simulink model "ensembleSNN_simulink"  (R2019a)
settings: Solver=FixedStepAuto  StartTime=0.0  StopTime=12  FixedStep=0.001  RelTol=1e-3
libraries: simulink x2, dspsigops x1
(part 1 of 3)
settings Model: Creator=40129232  LastModifiedBy=40175607
settings DataIOCC: ReturnWorkspaceOutputs=off
settings OptimizationCC: LifeSpan=inf
settings DebuggingCC: SFExecutionAtInitializationDiag=none  ArithmeticOperatorsInVariantConditions=warning
settings SFSimCC: SimUseLocalCustomCode=off
settings RTWCC: RTWUseLocalCustomCode=off
settings CodeAppCC: StateflowObjectComments=on

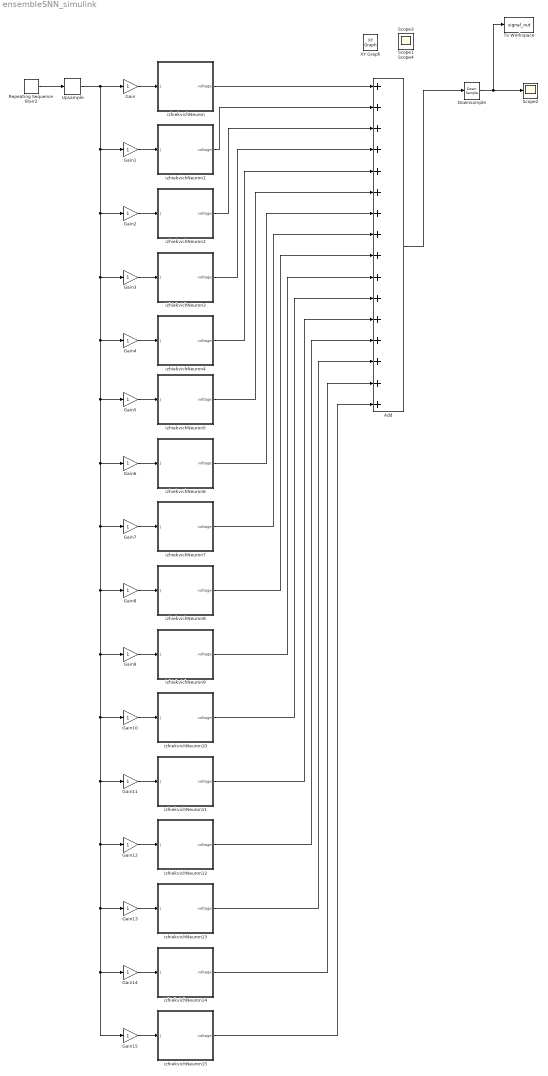
== system ensembleSNN_simulink ==
  Add : Sum  Inputs=++++++++++++++++
  Downsample : DownSample  N=12  phase=9  RateOptions=Allow multirate processing
  Gain{,1..15} (16 alike) : Gain
  Repeating Sequence Stair2 : simulink/Sources/Repeating Sequence Stair  OutValues=[40.37, 52.35, 62.17, 70.19, 76.75].'  tsamp=0.012  OutMin=[]  OutMax=[]  OutDataTypeStr=double  OutputDataTypeScalingMode=double  OutDataType=fixdt(0,8)  ConRadixGroup=Best Precision: Vector-wise  OutScaling=2^-12
  Scope{1..4} (4 alike) : Scope
  To Workspace : ToWorkspace  VariableName=signal_out  SampleTime=-1
  Upsample : dspsigops/Upsample  N=12  phase=0  RateOptions=Allow multirate processing  ic=0  mode=Unused parameter value
  izhiekvichNeuron : Subsystem
  izhiekvichNeuron1 : Subsystem
  izhiekvichNeuron10 : Subsystem
  izhiekvichNeuron11 : Subsystem
  izhiekvichNeuron12 : Subsystem
  izhiekvichNeuron13 : Subsystem
  izhiekvichNeuron14 : Subsystem
  izhiekvichNeuron15 : Subsystem
  izhiekvichNeuron2 : Subsystem
  izhiekvichNeuron3 : Subsystem
  izhiekvichNeuron4 : Subsystem
  izhiekvichNeuron5 : Subsystem
  izhiekvichNeuron6 : Subsystem
  izhiekvichNeuron7 : Subsystem
  izhiekvichNeuron8 : Subsystem
  izhiekvichNeuron9 : Subsystem
  XY Graph : simulink/Sinks/XY Graph  IOType=viewer  xmin=-1  xmax=1  ymin=-1  ymax=1  st=-1
  wires:
  Repeating Sequence Stair2/1 -> Upsample/1
  Downsample/1 -> To Workspace/1, Scope2/1
  Upsample/1 -> Gain3/1, Gain5/1, Gain6/1, Gain9/1, Gain11/1, Gain12/1, Gain15/1, Gain14/1, Gain13/1, Gain10/1, Gain8/1, Gain7/1, Gain4/1, Gain2/1, Gain1/1, Gain/1
  Gain/1 -> izhiekvichNeuron/1(J)
  Add/1 -> Downsample/1
  izhiekvichNeuron/1(voltage) -> Add/1
  izhiekvichNeuron15/1(voltage) -> Add/16
  izhiekvichNeuron14/1(voltage) -> Add/15
  izhiekvichNeuron13/1(voltage) -> Add/14
  izhiekvichNeuron12/1(voltage) -> Add/13
  izhiekvichNeuron11/1(voltage) -> Add/12
  izhiekvichNeuron10/1(voltage) -> Add/11
  izhiekvichNeuron9/1(voltage) -> Add/10
  izhiekvichNeuron8/1(voltage) -> Add/9
  izhiekvichNeuron7/1(voltage) -> Add/8
  izhiekvichNeuron6/1(voltage) -> Add/7
  izhiekvichNeuron5/1(voltage) -> Add/6
  izhiekvichNeuron4/1(voltage) -> Add/5
  izhiekvichNeuron3/1(voltage) -> Add/4
  izhiekvichNeuron2/1(voltage) -> Add/3
  izhiekvichNeuron1/1(voltage) -> Add/2
  Gain1/1 -> izhiekvichNeuron1/1(J)
  Gain2/1 -> izhiekvichNeuron2/1(J)
  Gain3/1 -> izhiekvichNeuron3/1(J)
  Gain4/1 -> izhiekvichNeuron4/1(J)
  Gain5/1 -> izhiekvichNeuron5/1(J)
  Gain6/1 -> izhiekvichNeuron6/1(J)
  Gain7/1 -> izhiekvichNeuron7/1(J)
  Gain8/1 -> izhiekvichNeuron8/1(J)
  Gain9/1 -> izhiekvichNeuron9/1(J)
  Gain10/1 -> izhiekvichNeuron10/1(J)
  Gain11/1 -> izhiekvichNeuron11/1(J)
  Gain12/1 -> izhiekvichNeuron12/1(J)
  Gain13/1 -> izhiekvichNeuron13/1(J)
  Gain14/1 -> izhiekvichNeuron14/1(J)
  Gain15/1 -> izhiekvichNeuron15/1(J)

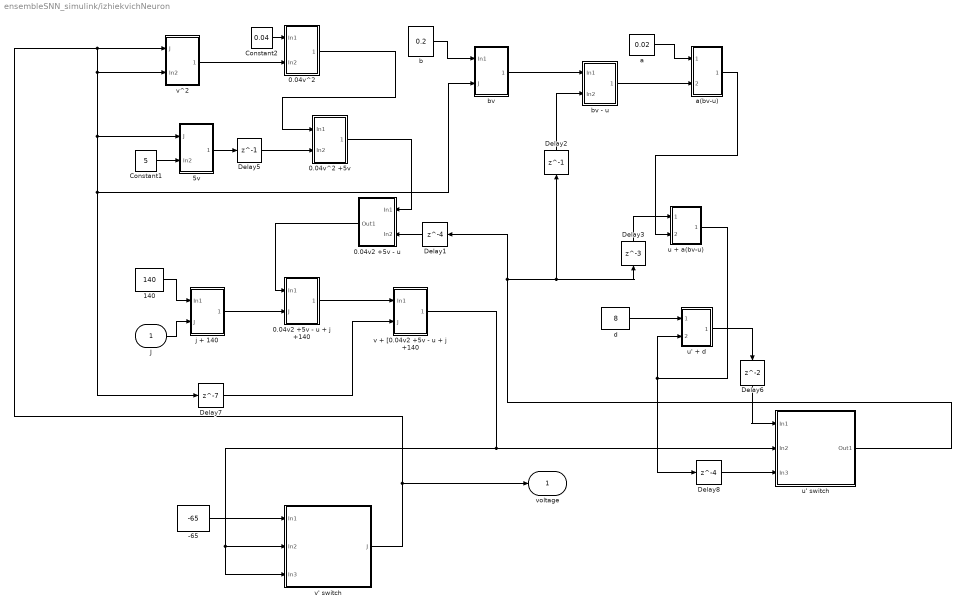
== system ensembleSNN_simulink/izhiekvichNeuron ==
  J : Inport
  -65 : Constant  Value=-65
  0.04v2 +5v - u : Subsystem
  0.04v2 +5v - u + j +140 : Subsystem
  0.04v^2 : Subsystem
  0.04v^2 +5v : Subsystem
  140 : Constant  Value=140
  5v : Subsystem
  Constant1 : Constant  Value=5
  Constant2 : Constant  Value=0.04
  Delay1 : Delay  DelayLength=4
  Delay2 : Delay  DelayLength=1
  Delay3 : Delay  DelayLength=3
  Delay5 : Delay  DelayLength=1
  Delay6 : Delay
  Delay7 : Delay  DelayLength=7
  Delay8 : Delay  DelayLength=4
  a : Constant  Value=0.02
  a(bv-u) : Subsystem
  b : Constant  Value=0.2
  bv : Subsystem
  bv - u : Subsystem
  d : Constant  Value=8
  j + 140 : Subsystem
  u + a(bv-u) : Subsystem
  u' + d : Subsystem
  u' switch : Subsystem
  v + [0.04v2 +5v - u + j +140 : Subsystem
  v' switch : Subsystem
  v^2 : Subsystem
  voltage : Outport
  wires:
  d/1 -> u' + d/1(In1)
  Constant1/1 -> 5v/2(In2)
  Constant2/1 -> 0.04v^2/1(In1)
  140/1 -> j + 140/1(In1)
  -65/1 -> v' switch/1(In1)
  b/1 -> bv/1(In1)
  a/1 -> a(bv-u)/1(In1)
  5v/1(Out1) -> Delay5/1
  J/1 -> j + 140/2(J)
  j + 140/1(Out1) -> 0.04v2 +5v - u + j +140/2(J)
  u' + d/1(Out1) -> Delay6/1
  u' switch/1(Out1) -> Delay1/1, Delay3/1, Delay2/1
  Delay1/1 -> 0.04v2 +5v - u/2(In2)
  Delay2/1 -> bv - u/2(In2)
  Delay3/1 -> u + a(bv-u)/1(In1)
  v' switch/1(J) -> v^2/1(J), v^2/2(In2), 5v/1(J), bv/2(J), Delay7/1, voltage/1
  Delay7/1 -> v + [0.04v2 +5v - u + j +140/2(J)
  v^2/1(Out1) -> 0.04v^2/2(In2)
  Delay5/1 -> 0.04v^2 +5v/2(In2)
  bv/1(Out1) -> bv - u/1(In1)
  0.04v^2/1(Out1) -> 0.04v^2 +5v/1(In1)
  bv - u/1(Out1) -> a(bv-u)/2(In2)
  0.04v^2 +5v/1(Out1) -> 0.04v2 +5v - u/1(In1)
  0.04v2 +5v - u/1(Out1) -> 0.04v2 +5v - u + j +140/1(In1)
  0.04v2 +5v - u + j +140/1(Out1) -> v + [0.04v2 +5v - u + j +140/1(In1)
  v + [0.04v2 +5v - u + j +140/1(Out1) -> u' switch/2(In2), v' switch/3(In3), v' switch/2(In2)
  a(bv-u)/1(Out1) -> u + a(bv-u)/2(In2)
  u + a(bv-u)/1(Out1) -> u' + d/2(In2), Delay8/1
  Delay8/1 -> u' switch/3(In3)
  Delay6/1 -> u' switch/1(In1)

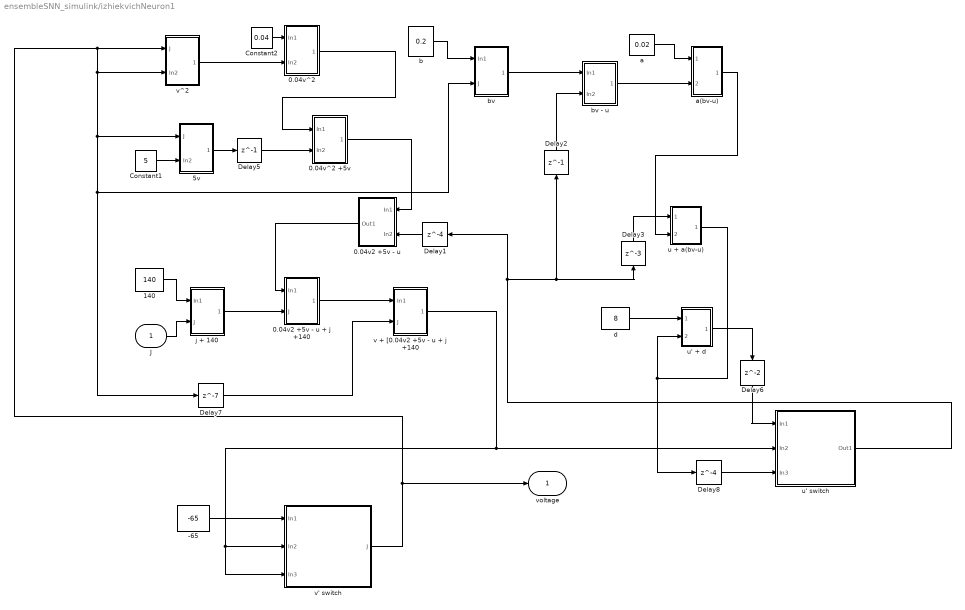
== system ensembleSNN_simulink/izhiekvichNeuron1 ==
  J : Inport
  -65 : Constant  Value=-65
  0.04v2 +5v - u : Subsystem
  0.04v2 +5v - u + j +140 : Subsystem
  0.04v^2 : Subsystem
  0.04v^2 +5v : Subsystem
  140 : Constant  Value=140
  5v : Subsystem
  Constant1 : Constant  Value=5
  Constant2 : Constant  Value=0.04
  Delay1 : Delay  DelayLength=4
  Delay2 : Delay  DelayLength=1
  Delay3 : Delay  DelayLength=3
  Delay5 : Delay  DelayLength=1
  Delay6 : Delay
  Delay7 : Delay  DelayLength=7
  Delay8 : Delay  DelayLength=4
  a : Constant  Value=0.02
  a(bv-u) : Subsystem
  b : Constant  Value=0.2
  bv : Subsystem
  bv - u : Subsystem
  d : Constant  Value=8
  j + 140 : Subsystem
  u + a(bv-u) : Subsystem
  u' + d : Subsystem
  u' switch : Subsystem
  v + [0.04v2 +5v - u + j +140 : Subsystem
  v' switch : Subsystem
  v^2 : Subsystem
  voltage : Outport
  wires:
  d/1 -> u' + d/1(In1)
  Constant1/1 -> 5v/2(In2)
  Constant2/1 -> 0.04v^2/1(In1)
  140/1 -> j + 140/1(In1)
  -65/1 -> v' switch/1(In1)
  b/1 -> bv/1(In1)
  a/1 -> a(bv-u)/1(In1)
  5v/1(Out1) -> Delay5/1
  J/1 -> j + 140/2(J)
  j + 140/1(Out1) -> 0.04v2 +5v - u + j +140/2(J)
  u' + d/1(Out1) -> Delay6/1
  u' switch/1(Out1) -> Delay1/1, Delay3/1, Delay2/1
  Delay1/1 -> 0.04v2 +5v - u/2(In2)
  Delay2/1 -> bv - u/2(In2)
  Delay3/1 -> u + a(bv-u)/1(In1)
  v' switch/1(J) -> v^2/1(J), v^2/2(In2), 5v/1(J), bv/2(J), Delay7/1, voltage/1
  Delay7/1 -> v + [0.04v2 +5v - u + j +140/2(J)
  v^2/1(Out1) -> 0.04v^2/2(In2)
  Delay5/1 -> 0.04v^2 +5v/2(In2)
  bv/1(Out1) -> bv - u/1(In1)
  0.04v^2/1(Out1) -> 0.04v^2 +5v/1(In1)
  bv - u/1(Out1) -> a(bv-u)/2(In2)
  0.04v^2 +5v/1(Out1) -> 0.04v2 +5v - u/1(In1)
  0.04v2 +5v - u/1(Out1) -> 0.04v2 +5v - u + j +140/1(In1)
  0.04v2 +5v - u + j +140/1(Out1) -> v + [0.04v2 +5v - u + j +140/1(In1)
  v + [0.04v2 +5v - u + j +140/1(Out1) -> u' switch/2(In2), v' switch/3(In3), v' switch/2(In2)
  a(bv-u)/1(Out1) -> u + a(bv-u)/2(In2)
  u + a(bv-u)/1(Out1) -> u' + d/2(In2), Delay8/1
  Delay8/1 -> u' switch/3(In3)
  Delay6/1 -> u' switch/1(In1)

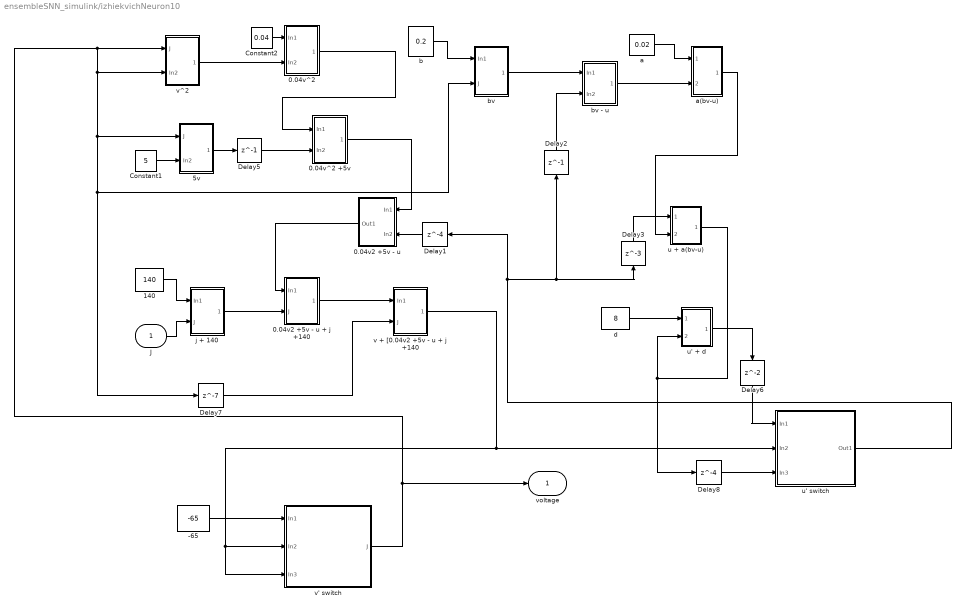
== system ensembleSNN_simulink/izhiekvichNeuron10 ==
  J : Inport
  -65 : Constant  Value=-65
  0.04v2 +5v - u : Subsystem
  0.04v2 +5v - u + j +140 : Subsystem
  0.04v^2 : Subsystem
  0.04v^2 +5v : Subsystem
  140 : Constant  Value=140
  5v : Subsystem
  Constant1 : Constant  Value=5
  Constant2 : Constant  Value=0.04
  Delay1 : Delay  DelayLength=4
  Delay2 : Delay  DelayLength=1
  Delay3 : Delay  DelayLength=3
  Delay5 : Delay  DelayLength=1
  Delay6 : Delay
  Delay7 : Delay  DelayLength=7
  Delay8 : Delay  DelayLength=4
  a : Constant  Value=0.02
  a(bv-u) : Subsystem
  b : Constant  Value=0.2
  bv : Subsystem
  bv - u : Subsystem
  d : Constant  Value=8
  j + 140 : Subsystem
  u + a(bv-u) : Subsystem
  u' + d : Subsystem
  u' switch : Subsystem
  v + [0.04v2 +5v - u + j +140 : Subsystem
  v' switch : Subsystem
  v^2 : Subsystem
  voltage : Outport
  wires:
  d/1 -> u' + d/1(In1)
  Constant1/1 -> 5v/2(In2)
  Constant2/1 -> 0.04v^2/1(In1)
  140/1 -> j + 140/1(In1)
  -65/1 -> v' switch/1(In1)
  b/1 -> bv/1(In1)
  a/1 -> a(bv-u)/1(In1)
  5v/1(Out1) -> Delay5/1
  J/1 -> j + 140/2(J)
  j + 140/1(Out1) -> 0.04v2 +5v - u + j +140/2(J)
  u' + d/1(Out1) -> Delay6/1
  u' switch/1(Out1) -> Delay1/1, Delay3/1, Delay2/1
  Delay1/1 -> 0.04v2 +5v - u/2(In2)
  Delay2/1 -> bv - u/2(In2)
  Delay3/1 -> u + a(bv-u)/1(In1)
  v' switch/1(J) -> v^2/1(J), v^2/2(In2), 5v/1(J), bv/2(J), Delay7/1, voltage/1
  Delay7/1 -> v + [0.04v2 +5v - u + j +140/2(J)
  v^2/1(Out1) -> 0.04v^2/2(In2)
  Delay5/1 -> 0.04v^2 +5v/2(In2)
  bv/1(Out1) -> bv - u/1(In1)
  0.04v^2/1(Out1) -> 0.04v^2 +5v/1(In1)
  bv - u/1(Out1) -> a(bv-u)/2(In2)
  0.04v^2 +5v/1(Out1) -> 0.04v2 +5v - u/1(In1)
  0.04v2 +5v - u/1(Out1) -> 0.04v2 +5v - u + j +140/1(In1)
  0.04v2 +5v - u + j +140/1(Out1) -> v + [0.04v2 +5v - u + j +140/1(In1)
  v + [0.04v2 +5v - u + j +140/1(Out1) -> u' switch/2(In2), v' switch/3(In3), v' switch/2(In2)
  a(bv-u)/1(Out1) -> u + a(bv-u)/2(In2)
  u + a(bv-u)/1(Out1) -> u' + d/2(In2), Delay8/1
  Delay8/1 -> u' switch/3(In3)
  Delay6/1 -> u' switch/1(In1)

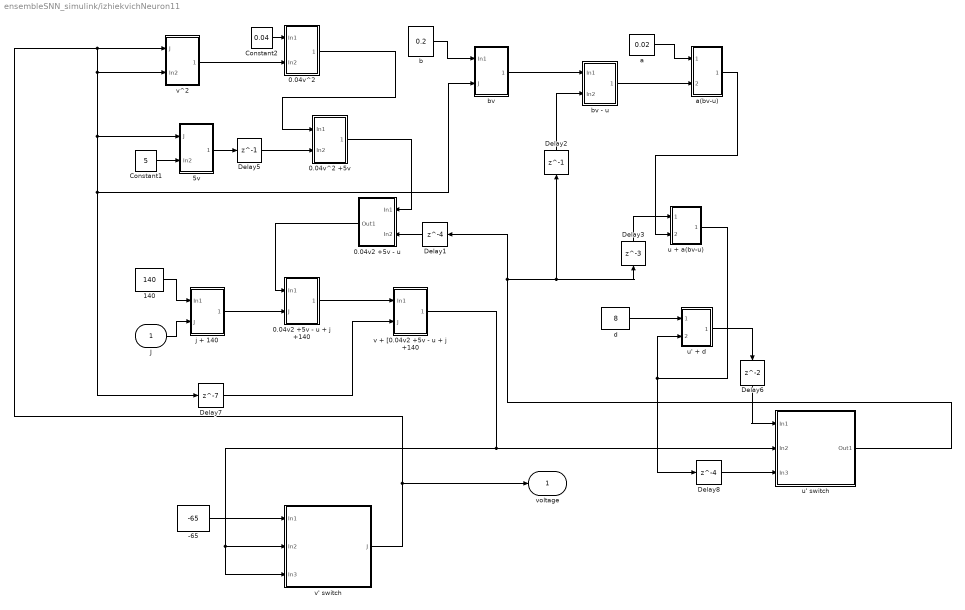
== system ensembleSNN_simulink/izhiekvichNeuron11 ==
  J : Inport
  -65 : Constant  Value=-65
  0.04v2 +5v - u : Subsystem
  0.04v2 +5v - u + j +140 : Subsystem
  0.04v^2 : Subsystem
  0.04v^2 +5v : Subsystem
  140 : Constant  Value=140
  5v : Subsystem
  Constant1 : Constant  Value=5
  Constant2 : Constant  Value=0.04
  Delay1 : Delay  DelayLength=4
  Delay2 : Delay  DelayLength=1
  Delay3 : Delay  DelayLength=3
  Delay5 : Delay  DelayLength=1
  Delay6 : Delay
  Delay7 : Delay  DelayLength=7
  Delay8 : Delay  DelayLength=4
  a : Constant  Value=0.02
  a(bv-u) : Subsystem
  b : Constant  Value=0.2
  bv : Subsystem
  bv - u : Subsystem
  d : Constant  Value=8
  j + 140 : Subsystem
  u + a(bv-u) : Subsystem
  u' + d : Subsystem
  u' switch : Subsystem
  v + [0.04v2 +5v - u + j +140 : Subsystem
  v' switch : Subsystem
  v^2 : Subsystem
  voltage : Outport
  wires:
  d/1 -> u' + d/1(In1)
  Constant1/1 -> 5v/2(In2)
  Constant2/1 -> 0.04v^2/1(In1)
  140/1 -> j + 140/1(In1)
  -65/1 -> v' switch/1(In1)
  b/1 -> bv/1(In1)
  a/1 -> a(bv-u)/1(In1)
  5v/1(Out1) -> Delay5/1
  J/1 -> j + 140/2(J)
  j + 140/1(Out1) -> 0.04v2 +5v - u + j +140/2(J)
  u' + d/1(Out1) -> Delay6/1
  u' switch/1(Out1) -> Delay1/1, Delay3/1, Delay2/1
  Delay1/1 -> 0.04v2 +5v - u/2(In2)
  Delay2/1 -> bv - u/2(In2)
  Delay3/1 -> u + a(bv-u)/1(In1)
  v' switch/1(J) -> v^2/1(J), v^2/2(In2), 5v/1(J), bv/2(J), Delay7/1, voltage/1
  Delay7/1 -> v + [0.04v2 +5v - u + j +140/2(J)
  v^2/1(Out1) -> 0.04v^2/2(In2)
  Delay5/1 -> 0.04v^2 +5v/2(In2)
  bv/1(Out1) -> bv - u/1(In1)
  0.04v^2/1(Out1) -> 0.04v^2 +5v/1(In1)
  bv - u/1(Out1) -> a(bv-u)/2(In2)
  0.04v^2 +5v/1(Out1) -> 0.04v2 +5v - u/1(In1)
  0.04v2 +5v - u/1(Out1) -> 0.04v2 +5v - u + j +140/1(In1)
  0.04v2 +5v - u + j +140/1(Out1) -> v + [0.04v2 +5v - u + j +140/1(In1)
  v + [0.04v2 +5v - u + j +140/1(Out1) -> u' switch/2(In2), v' switch/3(In3), v' switch/2(In2)
  a(bv-u)/1(Out1) -> u + a(bv-u)/2(In2)
  u + a(bv-u)/1(Out1) -> u' + d/2(In2), Delay8/1
  Delay8/1 -> u' switch/3(In3)
  Delay6/1 -> u' switch/1(In1)

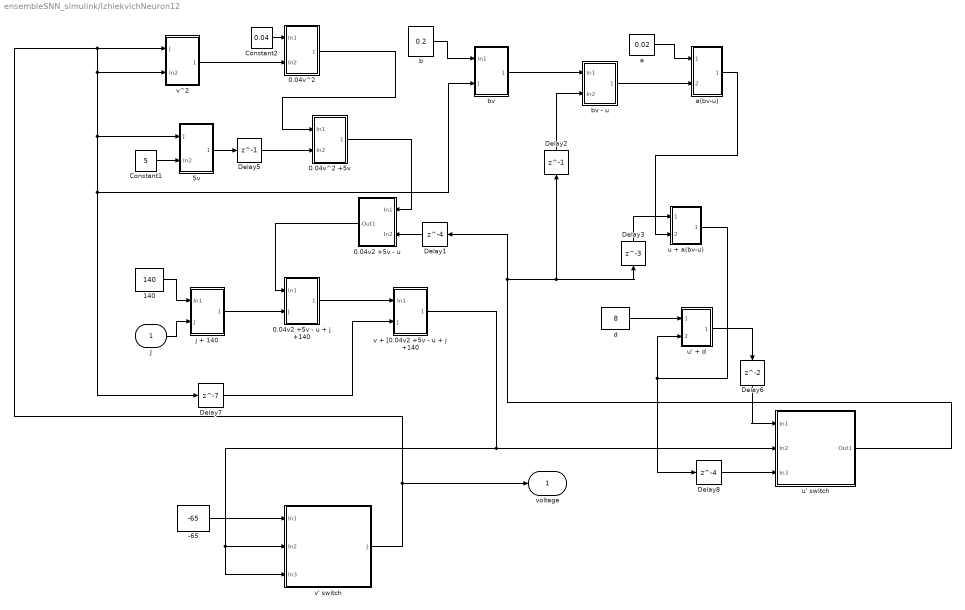
== system ensembleSNN_simulink/izhiekvichNeuron12 ==
  J : Inport
  -65 : Constant  Value=-65
  0.04v2 +5v - u : Subsystem
  0.04v2 +5v - u + j +140 : Subsystem
  0.04v^2 : Subsystem
  0.04v^2 +5v : Subsystem
  140 : Constant  Value=140
  5v : Subsystem
  Constant1 : Constant  Value=5
  Constant2 : Constant  Value=0.04
  Delay1 : Delay  DelayLength=4
  Delay2 : Delay  DelayLength=1
  Delay3 : Delay  DelayLength=3
  Delay5 : Delay  DelayLength=1
  Delay6 : Delay
  Delay7 : Delay  DelayLength=7
  Delay8 : Delay  DelayLength=4
  a : Constant  Value=0.02
  a(bv-u) : Subsystem
  b : Constant  Value=0.2
  bv : Subsystem
  bv - u : Subsystem
  d : Constant  Value=8
  j + 140 : Subsystem
  u + a(bv-u) : Subsystem
  u' + d : Subsystem
  u' switch : Subsystem
  v + [0.04v2 +5v - u + j +140 : Subsystem
  v' switch : Subsystem
  v^2 : Subsystem
  voltage : Outport
  wires:
  d/1 -> u' + d/1(In1)
  Constant1/1 -> 5v/2(In2)
  Constant2/1 -> 0.04v^2/1(In1)
  140/1 -> j + 140/1(In1)
  -65/1 -> v' switch/1(In1)
  b/1 -> bv/1(In1)
  a/1 -> a(bv-u)/1(In1)
  5v/1(Out1) -> Delay5/1
  J/1 -> j + 140/2(J)
  j + 140/1(Out1) -> 0.04v2 +5v - u + j +140/2(J)
  u' + d/1(Out1) -> Delay6/1
  u' switch/1(Out1) -> Delay1/1, Delay3/1, Delay2/1
  Delay1/1 -> 0.04v2 +5v - u/2(In2)
  Delay2/1 -> bv - u/2(In2)
  Delay3/1 -> u + a(bv-u)/1(In1)
  v' switch/1(J) -> v^2/1(J), v^2/2(In2), 5v/1(J), bv/2(J), Delay7/1, voltage/1
  Delay7/1 -> v + [0.04v2 +5v - u + j +140/2(J)
  v^2/1(Out1) -> 0.04v^2/2(In2)
  Delay5/1 -> 0.04v^2 +5v/2(In2)
  bv/1(Out1) -> bv - u/1(In1)
  0.04v^2/1(Out1) -> 0.04v^2 +5v/1(In1)
  bv - u/1(Out1) -> a(bv-u)/2(In2)
  0.04v^2 +5v/1(Out1) -> 0.04v2 +5v - u/1(In1)
  0.04v2 +5v - u/1(Out1) -> 0.04v2 +5v - u + j +140/1(In1)
  0.04v2 +5v - u + j +140/1(Out1) -> v + [0.04v2 +5v - u + j +140/1(In1)
  v + [0.04v2 +5v - u + j +140/1(Out1) -> u' switch/2(In2), v' switch/3(In3), v' switch/2(In2)
  a(bv-u)/1(Out1) -> u + a(bv-u)/2(In2)
  u + a(bv-u)/1(Out1) -> u' + d/2(In2), Delay8/1
  Delay8/1 -> u' switch/3(In3)
  Delay6/1 -> u' switch/1(In1)

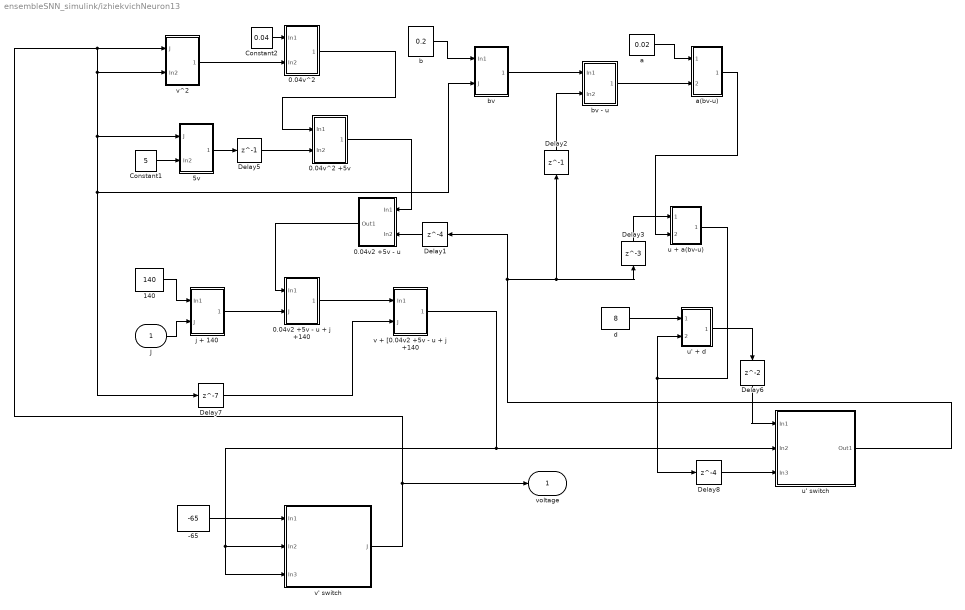
== system ensembleSNN_simulink/izhiekvichNeuron13 ==
  J : Inport
  -65 : Constant  Value=-65
  0.04v2 +5v - u : Subsystem
  0.04v2 +5v - u + j +140 : Subsystem
  0.04v^2 : Subsystem
  0.04v^2 +5v : Subsystem
  140 : Constant  Value=140
  5v : Subsystem
  Constant1 : Constant  Value=5
  Constant2 : Constant  Value=0.04
  Delay1 : Delay  DelayLength=4
  Delay2 : Delay  DelayLength=1
  Delay3 : Delay  DelayLength=3
  Delay5 : Delay  DelayLength=1
  Delay6 : Delay
  Delay7 : Delay  DelayLength=7
  Delay8 : Delay  DelayLength=4
  a : Constant  Value=0.02
  a(bv-u) : Subsystem
  b : Constant  Value=0.2
  bv : Subsystem
  bv - u : Subsystem
  d : Constant  Value=8
  j + 140 : Subsystem
  u + a(bv-u) : Subsystem
  u' + d : Subsystem
  u' switch : Subsystem
  v + [0.04v2 +5v - u + j +140 : Subsystem
  v' switch : Subsystem
  v^2 : Subsystem
  voltage : Outport
  wires:
  d/1 -> u' + d/1(In1)
  Constant1/1 -> 5v/2(In2)
  Constant2/1 -> 0.04v^2/1(In1)
  140/1 -> j + 140/1(In1)
  -65/1 -> v' switch/1(In1)
  b/1 -> bv/1(In1)
  a/1 -> a(bv-u)/1(In1)
  5v/1(Out1) -> Delay5/1
  J/1 -> j + 140/2(J)
  j + 140/1(Out1) -> 0.04v2 +5v - u + j +140/2(J)
  u' + d/1(Out1) -> Delay6/1
  u' switch/1(Out1) -> Delay1/1, Delay3/1, Delay2/1
  Delay1/1 -> 0.04v2 +5v - u/2(In2)
  Delay2/1 -> bv - u/2(In2)
  Delay3/1 -> u + a(bv-u)/1(In1)
  v' switch/1(J) -> v^2/1(J), v^2/2(In2), 5v/1(J), bv/2(J), Delay7/1, voltage/1
  Delay7/1 -> v + [0.04v2 +5v - u + j +140/2(J)
  v^2/1(Out1) -> 0.04v^2/2(In2)
  Delay5/1 -> 0.04v^2 +5v/2(In2)
  bv/1(Out1) -> bv - u/1(In1)
  0.04v^2/1(Out1) -> 0.04v^2 +5v/1(In1)
  bv - u/1(Out1) -> a(bv-u)/2(In2)
  0.04v^2 +5v/1(Out1) -> 0.04v2 +5v - u/1(In1)
  0.04v2 +5v - u/1(Out1) -> 0.04v2 +5v - u + j +140/1(In1)
  0.04v2 +5v - u + j +140/1(Out1) -> v + [0.04v2 +5v - u + j +140/1(In1)
  v + [0.04v2 +5v - u + j +140/1(Out1) -> u' switch/2(In2), v' switch/3(In3), v' switch/2(In2)
  a(bv-u)/1(Out1) -> u + a(bv-u)/2(In2)
  u + a(bv-u)/1(Out1) -> u' + d/2(In2), Delay8/1
  Delay8/1 -> u' switch/3(In3)
  Delay6/1 -> u' switch/1(In1)

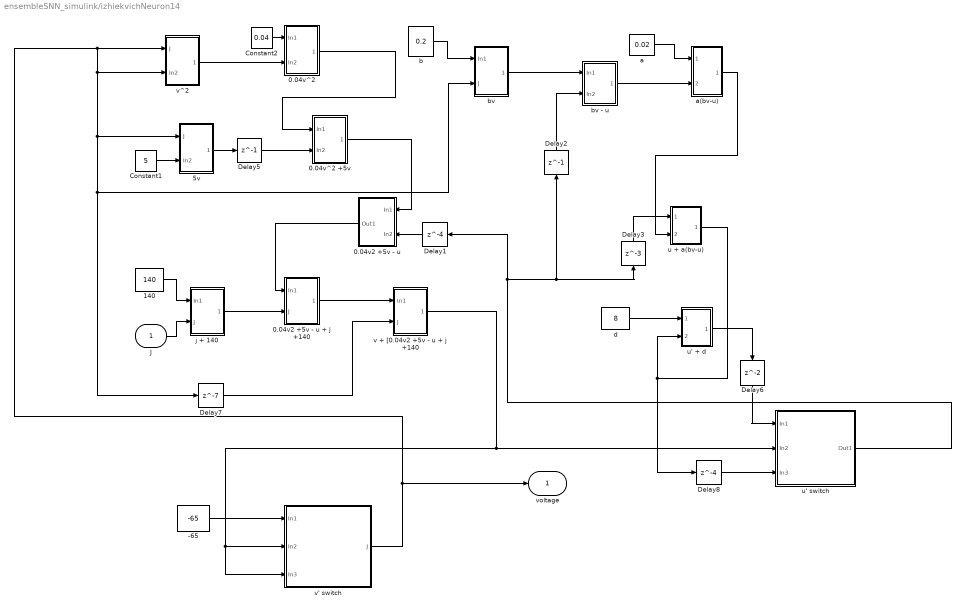
== system ensembleSNN_simulink/izhiekvichNeuron14 ==
  J : Inport
  -65 : Constant  Value=-65
  0.04v2 +5v - u : Subsystem
  0.04v2 +5v - u + j +140 : Subsystem
  0.04v^2 : Subsystem
  0.04v^2 +5v : Subsystem
  140 : Constant  Value=140
  5v : Subsystem
  Constant1 : Constant  Value=5
  Constant2 : Constant  Value=0.04
  Delay1 : Delay  DelayLength=4
  Delay2 : Delay  DelayLength=1
  Delay3 : Delay  DelayLength=3
  Delay5 : Delay  DelayLength=1
  Delay6 : Delay
  Delay7 : Delay  DelayLength=7
  Delay8 : Delay  DelayLength=4
  a : Constant  Value=0.02
  a(bv-u) : Subsystem
  b : Constant  Value=0.2
  bv : Subsystem
  bv - u : Subsystem
  d : Constant  Value=8
  j + 140 : Subsystem
  u + a(bv-u) : Subsystem
  u' + d : Subsystem
  u' switch : Subsystem
  v + [0.04v2 +5v - u + j +140 : Subsystem
  v' switch : Subsystem
  v^2 : Subsystem
  voltage : Outport
  wires:
  d/1 -> u' + d/1(In1)
  Constant1/1 -> 5v/2(In2)
  Constant2/1 -> 0.04v^2/1(In1)
  140/1 -> j + 140/1(In1)
  -65/1 -> v' switch/1(In1)
  b/1 -> bv/1(In1)
  a/1 -> a(bv-u)/1(In1)
  5v/1(Out1) -> Delay5/1
  J/1 -> j + 140/2(J)
  j + 140/1(Out1) -> 0.04v2 +5v - u + j +140/2(J)
  u' + d/1(Out1) -> Delay6/1
  u' switch/1(Out1) -> Delay1/1, Delay3/1, Delay2/1
  Delay1/1 -> 0.04v2 +5v - u/2(In2)
  Delay2/1 -> bv - u/2(In2)
  Delay3/1 -> u + a(bv-u)/1(In1)
  v' switch/1(J) -> v^2/1(J), v^2/2(In2), 5v/1(J), bv/2(J), Delay7/1, voltage/1
  Delay7/1 -> v + [0.04v2 +5v - u + j +140/2(J)
  v^2/1(Out1) -> 0.04v^2/2(In2)
  Delay5/1 -> 0.04v^2 +5v/2(In2)
  bv/1(Out1) -> bv - u/1(In1)
  0.04v^2/1(Out1) -> 0.04v^2 +5v/1(In1)
  bv - u/1(Out1) -> a(bv-u)/2(In2)
  0.04v^2 +5v/1(Out1) -> 0.04v2 +5v - u/1(In1)
  0.04v2 +5v - u/1(Out1) -> 0.04v2 +5v - u + j +140/1(In1)
  0.04v2 +5v - u + j +140/1(Out1) -> v + [0.04v2 +5v - u + j +140/1(In1)
  v + [0.04v2 +5v - u + j +140/1(Out1) -> u' switch/2(In2), v' switch/3(In3), v' switch/2(In2)
  a(bv-u)/1(Out1) -> u + a(bv-u)/2(In2)
  u + a(bv-u)/1(Out1) -> u' + d/2(In2), Delay8/1
  Delay8/1 -> u' switch/3(In3)
  Delay6/1 -> u' switch/1(In1)

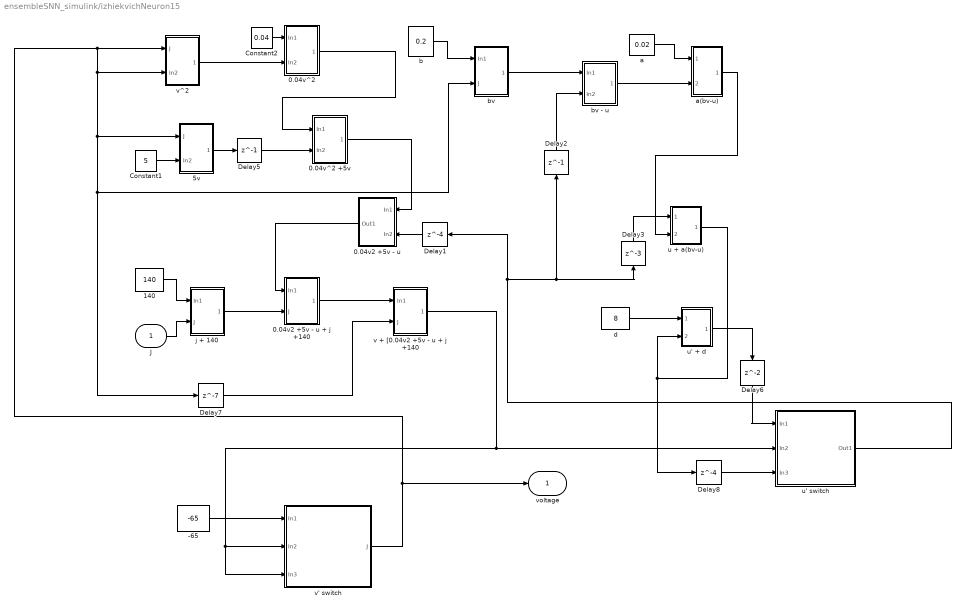
== system ensembleSNN_simulink/izhiekvichNeuron15 ==
  J : Inport
  -65 : Constant  Value=-65
  0.04v2 +5v - u : Subsystem
  0.04v2 +5v - u + j +140 : Subsystem
  0.04v^2 : Subsystem
  0.04v^2 +5v : Subsystem
  140 : Constant  Value=140
  5v : Subsystem
  Constant1 : Constant  Value=5
  Constant2 : Constant  Value=0.04
  Delay1 : Delay  DelayLength=4
  Delay2 : Delay  DelayLength=1
  Delay3 : Delay  DelayLength=3
  Delay5 : Delay  DelayLength=1
  Delay6 : Delay
  Delay7 : Delay  DelayLength=7
  Delay8 : Delay  DelayLength=4
  a : Constant  Value=0.02
  a(bv-u) : Subsystem
  b : Constant  Value=0.2
  bv : Subsystem
  bv - u : Subsystem
  d : Constant  Value=8
  j + 140 : Subsystem
  u + a(bv-u) : Subsystem
  u' + d : Subsystem
  u' switch : Subsystem
  v + [0.04v2 +5v - u + j +140 : Subsystem
  v' switch : Subsystem
  v^2 : Subsystem
  voltage : Outport
  wires:
  d/1 -> u' + d/1(In1)
  Constant1/1 -> 5v/2(In2)
  Constant2/1 -> 0.04v^2/1(In1)
  140/1 -> j + 140/1(In1)
  -65/1 -> v' switch/1(In1)
  b/1 -> bv/1(In1)
  a/1 -> a(bv-u)/1(In1)
  5v/1(Out1) -> Delay5/1
  J/1 -> j + 140/2(J)
  j + 140/1(Out1) -> 0.04v2 +5v - u + j +140/2(J)
  u' + d/1(Out1) -> Delay6/1
  u' switch/1(Out1) -> Delay1/1, Delay3/1, Delay2/1
  Delay1/1 -> 0.04v2 +5v - u/2(In2)
  Delay2/1 -> bv - u/2(In2)
  Delay3/1 -> u + a(bv-u)/1(In1)
  v' switch/1(J) -> v^2/1(J), v^2/2(In2), 5v/1(J), bv/2(J), Delay7/1, voltage/1
  Delay7/1 -> v + [0.04v2 +5v - u + j +140/2(J)
  v^2/1(Out1) -> 0.04v^2/2(In2)
  Delay5/1 -> 0.04v^2 +5v/2(In2)
  bv/1(Out1) -> bv - u/1(In1)
  0.04v^2/1(Out1) -> 0.04v^2 +5v/1(In1)
  bv - u/1(Out1) -> a(bv-u)/2(In2)
  0.04v^2 +5v/1(Out1) -> 0.04v2 +5v - u/1(In1)
  0.04v2 +5v - u/1(Out1) -> 0.04v2 +5v - u + j +140/1(In1)
  0.04v2 +5v - u + j +140/1(Out1) -> v + [0.04v2 +5v - u + j +140/1(In1)
  v + [0.04v2 +5v - u + j +140/1(Out1) -> u' switch/2(In2), v' switch/3(In3), v' switch/2(In2)
  a(bv-u)/1(Out1) -> u + a(bv-u)/2(In2)
  u + a(bv-u)/1(Out1) -> u' + d/2(In2), Delay8/1
  Delay8/1 -> u' switch/3(In3)
  Delay6/1 -> u' switch/1(In1)

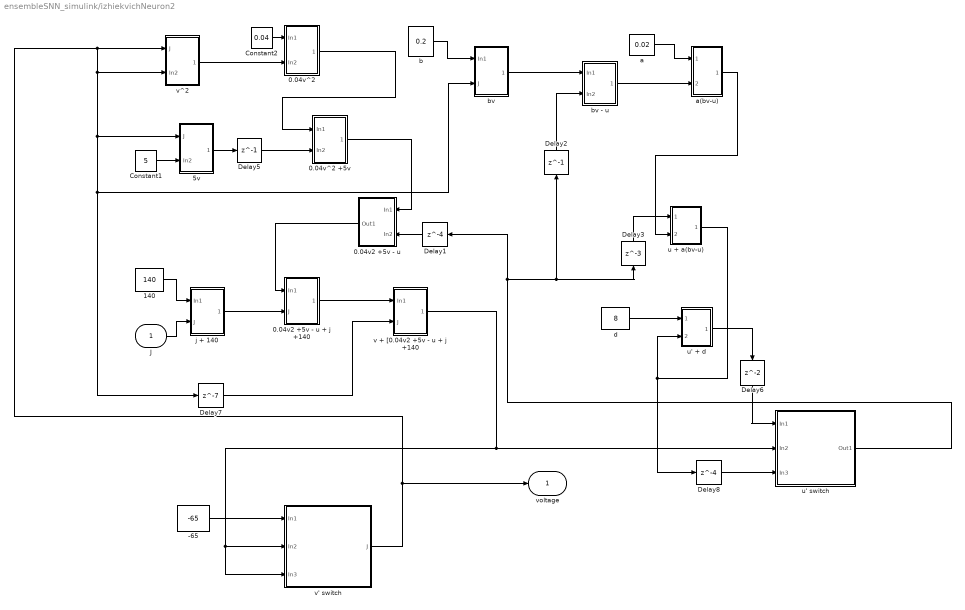
== system ensembleSNN_simulink/izhiekvichNeuron2 ==
  J : Inport
  -65 : Constant  Value=-65
  0.04v2 +5v - u : Subsystem
  0.04v2 +5v - u + j +140 : Subsystem
  0.04v^2 : Subsystem
  0.04v^2 +5v : Subsystem
  140 : Constant  Value=140
  5v : Subsystem
  Constant1 : Constant  Value=5
  Constant2 : Constant  Value=0.04
  Delay1 : Delay  DelayLength=4
  Delay2 : Delay  DelayLength=1
  Delay3 : Delay  DelayLength=3
  Delay5 : Delay  DelayLength=1
  Delay6 : Delay
  Delay7 : Delay  DelayLength=7
  Delay8 : Delay  DelayLength=4
  a : Constant  Value=0.02
  a(bv-u) : Subsystem
  b : Constant  Value=0.2
  bv : Subsystem
  bv - u : Subsystem
  d : Constant  Value=8
  j + 140 : Subsystem
  u + a(bv-u) : Subsystem
  u' + d : Subsystem
  u' switch : Subsystem
  v + [0.04v2 +5v - u + j +140 : Subsystem
  v' switch : Subsystem
  v^2 : Subsystem
  voltage : Outport
  wires:
  d/1 -> u' + d/1(In1)
  Constant1/1 -> 5v/2(In2)
  Constant2/1 -> 0.04v^2/1(In1)
  140/1 -> j + 140/1(In1)
  -65/1 -> v' switch/1(In1)
  b/1 -> bv/1(In1)
  a/1 -> a(bv-u)/1(In1)
  5v/1(Out1) -> Delay5/1
  J/1 -> j + 140/2(J)
  j + 140/1(Out1) -> 0.04v2 +5v - u + j +140/2(J)
  u' + d/1(Out1) -> Delay6/1
  u' switch/1(Out1) -> Delay1/1, Delay3/1, Delay2/1
  Delay1/1 -> 0.04v2 +5v - u/2(In2)
  Delay2/1 -> bv - u/2(In2)
  Delay3/1 -> u + a(bv-u)/1(In1)
  v' switch/1(J) -> v^2/1(J), v^2/2(In2), 5v/1(J), bv/2(J), Delay7/1, voltage/1
  Delay7/1 -> v + [0.04v2 +5v - u + j +140/2(J)
  v^2/1(Out1) -> 0.04v^2/2(In2)
  Delay5/1 -> 0.04v^2 +5v/2(In2)
  bv/1(Out1) -> bv - u/1(In1)
  0.04v^2/1(Out1) -> 0.04v^2 +5v/1(In1)
  bv - u/1(Out1) -> a(bv-u)/2(In2)
  0.04v^2 +5v/1(Out1) -> 0.04v2 +5v - u/1(In1)
  0.04v2 +5v - u/1(Out1) -> 0.04v2 +5v - u + j +140/1(In1)
  0.04v2 +5v - u + j +140/1(Out1) -> v + [0.04v2 +5v - u + j +140/1(In1)
  v + [0.04v2 +5v - u + j +140/1(Out1) -> u' switch/2(In2), v' switch/3(In3), v' switch/2(In2)
  a(bv-u)/1(Out1) -> u + a(bv-u)/2(In2)
  u + a(bv-u)/1(Out1) -> u' + d/2(In2), Delay8/1
  Delay8/1 -> u' switch/3(In3)
  Delay6/1 -> u' switch/1(In1)

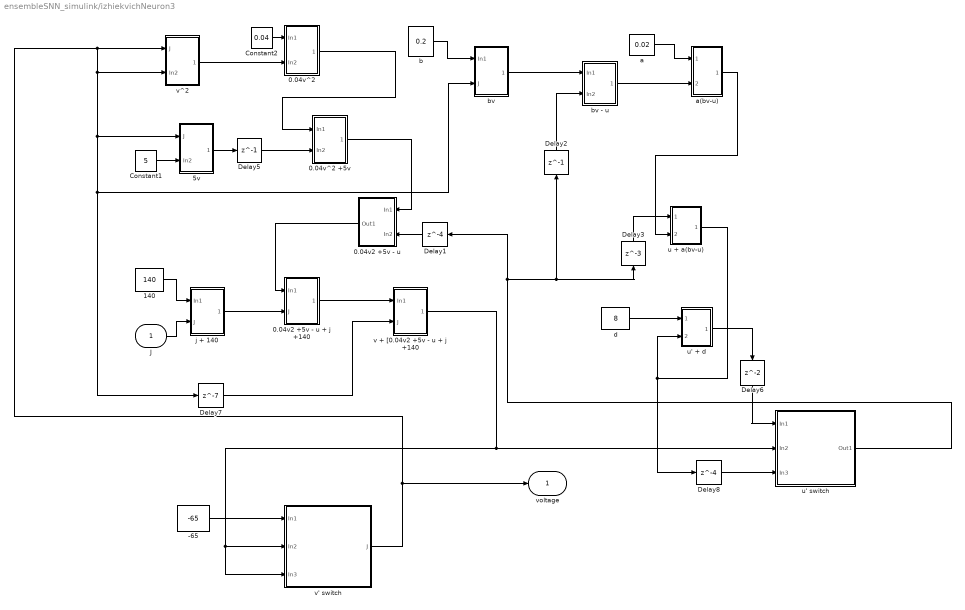
== system ensembleSNN_simulink/izhiekvichNeuron3 ==
  J : Inport
  -65 : Constant  Value=-65
  0.04v2 +5v - u : Subsystem
  0.04v2 +5v - u + j +140 : Subsystem
  0.04v^2 : Subsystem
  0.04v^2 +5v : Subsystem
  140 : Constant  Value=140
  5v : Subsystem
  Constant1 : Constant  Value=5
  Constant2 : Constant  Value=0.04
  Delay1 : Delay  DelayLength=4
  Delay2 : Delay  DelayLength=1
  Delay3 : Delay  DelayLength=3
  Delay5 : Delay  DelayLength=1
  Delay6 : Delay
  Delay7 : Delay  DelayLength=7
  Delay8 : Delay  DelayLength=4
  a : Constant  Value=0.02
  a(bv-u) : Subsystem
  b : Constant  Value=0.2
  bv : Subsystem
  bv - u : Subsystem
  d : Constant  Value=8
  j + 140 : Subsystem
  u + a(bv-u) : Subsystem
  u' + d : Subsystem
  u' switch : Subsystem
  v + [0.04v2 +5v - u + j +140 : Subsystem
  v' switch : Subsystem
  v^2 : Subsystem
  voltage : Outport
  wires:
  d/1 -> u' + d/1(In1)
  Constant1/1 -> 5v/2(In2)
  Constant2/1 -> 0.04v^2/1(In1)
  140/1 -> j + 140/1(In1)
  -65/1 -> v' switch/1(In1)
  b/1 -> bv/1(In1)
  a/1 -> a(bv-u)/1(In1)
  5v/1(Out1) -> Delay5/1
  J/1 -> j + 140/2(J)
  j + 140/1(Out1) -> 0.04v2 +5v - u + j +140/2(J)
  u' + d/1(Out1) -> Delay6/1
  u' switch/1(Out1) -> Delay1/1, Delay3/1, Delay2/1
  Delay1/1 -> 0.04v2 +5v - u/2(In2)
  Delay2/1 -> bv - u/2(In2)
  Delay3/1 -> u + a(bv-u)/1(In1)
  v' switch/1(J) -> v^2/1(J), v^2/2(In2), 5v/1(J), bv/2(J), Delay7/1, voltage/1
  Delay7/1 -> v + [0.04v2 +5v - u + j +140/2(J)
  v^2/1(Out1) -> 0.04v^2/2(In2)
  Delay5/1 -> 0.04v^2 +5v/2(In2)
  bv/1(Out1) -> bv - u/1(In1)
  0.04v^2/1(Out1) -> 0.04v^2 +5v/1(In1)
  bv - u/1(Out1) -> a(bv-u)/2(In2)
  0.04v^2 +5v/1(Out1) -> 0.04v2 +5v - u/1(In1)
  0.04v2 +5v - u/1(Out1) -> 0.04v2 +5v - u + j +140/1(In1)
  0.04v2 +5v - u + j +140/1(Out1) -> v + [0.04v2 +5v - u + j +140/1(In1)
  v + [0.04v2 +5v - u + j +140/1(Out1) -> u' switch/2(In2), v' switch/3(In3), v' switch/2(In2)
  a(bv-u)/1(Out1) -> u + a(bv-u)/2(In2)
  u + a(bv-u)/1(Out1) -> u' + d/2(In2), Delay8/1
  Delay8/1 -> u' switch/3(In3)
  Delay6/1 -> u' switch/1(In1)

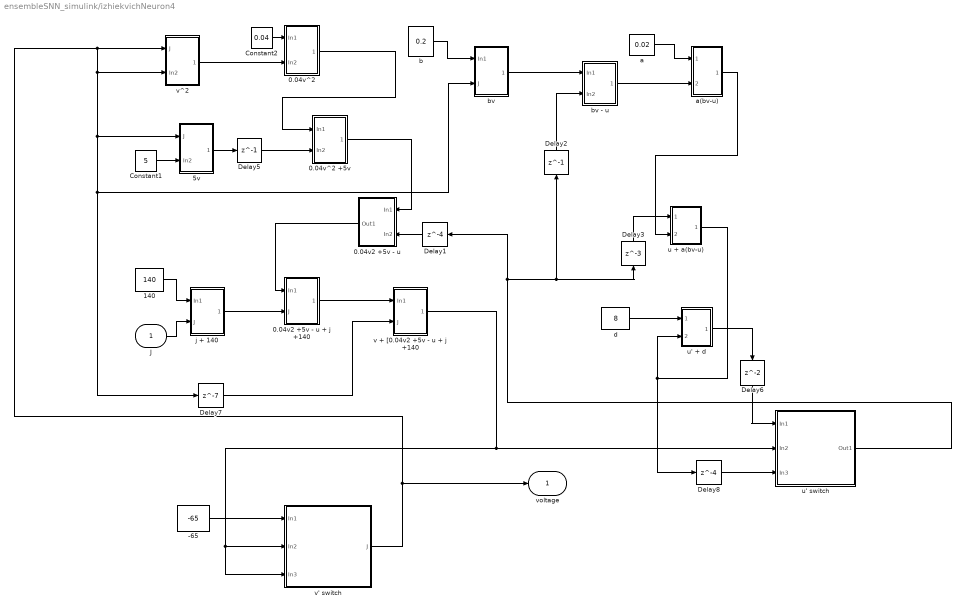
== system ensembleSNN_simulink/izhiekvichNeuron4 ==
  J : Inport
  -65 : Constant  Value=-65
  0.04v2 +5v - u : Subsystem
  0.04v2 +5v - u + j +140 : Subsystem
  0.04v^2 : Subsystem
  0.04v^2 +5v : Subsystem
  140 : Constant  Value=140
  5v : Subsystem
  Constant1 : Constant  Value=5
  Constant2 : Constant  Value=0.04
  Delay1 : Delay  DelayLength=4
  Delay2 : Delay  DelayLength=1
  Delay3 : Delay  DelayLength=3
  Delay5 : Delay  DelayLength=1
  Delay6 : Delay
  Delay7 : Delay  DelayLength=7
  Delay8 : Delay  DelayLength=4
  a : Constant  Value=0.02
  a(bv-u) : Subsystem
  b : Constant  Value=0.2
  bv : Subsystem
  bv - u : Subsystem
  d : Constant  Value=8
  j + 140 : Subsystem
  u + a(bv-u) : Subsystem
  u' + d : Subsystem
  u' switch : Subsystem
  v + [0.04v2 +5v - u + j +140 : Subsystem
  v' switch : Subsystem
  v^2 : Subsystem
  voltage : Outport
  wires:
  d/1 -> u' + d/1(In1)
  Constant1/1 -> 5v/2(In2)
  Constant2/1 -> 0.04v^2/1(In1)
  140/1 -> j + 140/1(In1)
  -65/1 -> v' switch/1(In1)
  b/1 -> bv/1(In1)
  a/1 -> a(bv-u)/1(In1)
  5v/1(Out1) -> Delay5/1
  J/1 -> j + 140/2(J)
  j + 140/1(Out1) -> 0.04v2 +5v - u + j +140/2(J)
  u' + d/1(Out1) -> Delay6/1
  u' switch/1(Out1) -> Delay1/1, Delay3/1, Delay2/1
  Delay1/1 -> 0.04v2 +5v - u/2(In2)
  Delay2/1 -> bv - u/2(In2)
  Delay3/1 -> u + a(bv-u)/1(In1)
  v' switch/1(J) -> v^2/1(J), v^2/2(In2), 5v/1(J), bv/2(J), Delay7/1, voltage/1
  Delay7/1 -> v + [0.04v2 +5v - u + j +140/2(J)
  v^2/1(Out1) -> 0.04v^2/2(In2)
  Delay5/1 -> 0.04v^2 +5v/2(In2)
  bv/1(Out1) -> bv - u/1(In1)
  0.04v^2/1(Out1) -> 0.04v^2 +5v/1(In1)
  bv - u/1(Out1) -> a(bv-u)/2(In2)
  0.04v^2 +5v/1(Out1) -> 0.04v2 +5v - u/1(In1)
  0.04v2 +5v - u/1(Out1) -> 0.04v2 +5v - u + j +140/1(In1)
  0.04v2 +5v - u + j +140/1(Out1) -> v + [0.04v2 +5v - u + j +140/1(In1)
  v + [0.04v2 +5v - u + j +140/1(Out1) -> u' switch/2(In2), v' switch/3(In3), v' switch/2(In2)
  a(bv-u)/1(Out1) -> u + a(bv-u)/2(In2)
  u + a(bv-u)/1(Out1) -> u' + d/2(In2), Delay8/1
  Delay8/1 -> u' switch/3(In3)
  Delay6/1 -> u' switch/1(In1)

== system ensembleSNN_simulink/izhiekvichNeuron5 ==
  J : Inport
  -65 : Constant  Value=-65
  0.04v2 +5v - u : Subsystem
  0.04v2 +5v - u + j +140 : Subsystem
  0.04v^2 : Subsystem
  0.04v^2 +5v : Subsystem
  140 : Constant  Value=140
  5v : Subsystem
  Constant1 : Constant  Value=5
  Constant2 : Constant  Value=0.04
  Delay1 : Delay  DelayLength=4
  Delay2 : Delay  DelayLength=1
  Delay3 : Delay  DelayLength=3
  Delay5 : Delay  DelayLength=1
  Delay6 : Delay
  Delay7 : Delay  DelayLength=7
  Delay8 : Delay  DelayLength=4
  a : Constant  Value=0.02
  a(bv-u) : Subsystem
  b : Constant  Value=0.2
  bv : Subsystem
  bv - u : Subsystem
  d : Constant  Value=8
  j + 140 : Subsystem
  u + a(bv-u) : Subsystem
  u' + d : Subsystem
  u' switch : Subsystem
  v + [0.04v2 +5v - u + j +140 : Subsystem
  v' switch : Subsystem
  v^2 : Subsystem
  voltage : Outport
  wires:
  d/1 -> u' + d/1(In1)
  Constant1/1 -> 5v/2(In2)
  Constant2/1 -> 0.04v^2/1(In1)
  140/1 -> j + 140/1(In1)
  -65/1 -> v' switch/1(In1)
  b/1 -> bv/1(In1)
  a/1 -> a(bv-u)/1(In1)
  5v/1(Out1) -> Delay5/1
  J/1 -> j + 140/2(J)
  j + 140/1(Out1) -> 0.04v2 +5v - u + j +140/2(J)
  u' + d/1(Out1) -> Delay6/1
  u' switch/1(Out1) -> Delay1/1, Delay3/1, Delay2/1
  Delay1/1 -> 0.04v2 +5v - u/2(In2)
  Delay2/1 -> bv - u/2(In2)
  Delay3/1 -> u + a(bv-u)/1(In1)
  v' switch/1(J) -> v^2/1(J), v^2/2(In2), 5v/1(J), bv/2(J), Delay7/1, voltage/1
  Delay7/1 -> v + [0.04v2 +5v - u + j +140/2(J)
  v^2/1(Out1) -> 0.04v^2/2(In2)
  Delay5/1 -> 0.04v^2 +5v/2(In2)
  bv/1(Out1) -> bv - u/1(In1)
  0.04v^2/1(Out1) -> 0.04v^2 +5v/1(In1)
  bv - u/1(Out1) -> a(bv-u)/2(In2)
  0.04v^2 +5v/1(Out1) -> 0.04v2 +5v - u/1(In1)
  0.04v2 +5v - u/1(Out1) -> 0.04v2 +5v - u + j +140/1(In1)
  0.04v2 +5v - u + j +140/1(Out1) -> v + [0.04v2 +5v - u + j +140/1(In1)
  v + [0.04v2 +5v - u + j +140/1(Out1) -> u' switch/2(In2), v' switch/3(In3), v' switch/2(In2)
  a(bv-u)/1(Out1) -> u + a(bv-u)/2(In2)
  u + a(bv-u)/1(Out1) -> u' + d/2(In2), Delay8/1
  Delay8/1 -> u' switch/3(In3)
  Delay6/1 -> u' switch/1(In1)

== system ensembleSNN_simulink/izhiekvichNeuron6 ==
  J : Inport
  -65 : Constant  Value=-65
  0.04v2 +5v - u : Subsystem
  0.04v2 +5v - u + j +140 : Subsystem
  0.04v^2 : Subsystem
  0.04v^2 +5v : Subsystem
  140 : Constant  Value=140
  5v : Subsystem
  Constant1 : Constant  Value=5
  Constant2 : Constant  Value=0.04
  Delay1 : Delay  DelayLength=4
  Delay2 : Delay  DelayLength=1
  Delay3 : Delay  DelayLength=3
  Delay5 : Delay  DelayLength=1
  Delay6 : Delay
  Delay7 : Delay  DelayLength=7
  Delay8 : Delay  DelayLength=4
  a : Constant  Value=0.02
  a(bv-u) : Subsystem
  b : Constant  Value=0.2
  bv : Subsystem
  bv - u : Subsystem
  d : Constant  Value=8
  j + 140 : Subsystem
  u + a(bv-u) : Subsystem
  u' + d : Subsystem
  u' switch : Subsystem
  v + [0.04v2 +5v - u + j +140 : Subsystem
  v' switch : Subsystem
  v^2 : Subsystem
  voltage : Outport
  wires:
  d/1 -> u' + d/1(In1)
  Constant1/1 -> 5v/2(In2)
  Constant2/1 -> 0.04v^2/1(In1)
  140/1 -> j + 140/1(In1)
  -65/1 -> v' switch/1(In1)
  b/1 -> bv/1(In1)
  a/1 -> a(bv-u)/1(In1)
  5v/1(Out1) -> Delay5/1
  J/1 -> j + 140/2(J)
  j + 140/1(Out1) -> 0.04v2 +5v - u + j +140/2(J)
  u' + d/1(Out1) -> Delay6/1
  u' switch/1(Out1) -> Delay1/1, Delay3/1, Delay2/1
  Delay1/1 -> 0.04v2 +5v - u/2(In2)
  Delay2/1 -> bv - u/2(In2)
  Delay3/1 -> u + a(bv-u)/1(In1)
  v' switch/1(J) -> v^2/1(J), v^2/2(In2), 5v/1(J), bv/2(J), Delay7/1, voltage/1
  Delay7/1 -> v + [0.04v2 +5v - u + j +140/2(J)
  v^2/1(Out1) -> 0.04v^2/2(In2)
  Delay5/1 -> 0.04v^2 +5v/2(In2)
  bv/1(Out1) -> bv - u/1(In1)
  0.04v^2/1(Out1) -> 0.04v^2 +5v/1(In1)
  bv - u/1(Out1) -> a(bv-u)/2(In2)
  0.04v^2 +5v/1(Out1) -> 0.04v2 +5v - u/1(In1)
  0.04v2 +5v - u/1(Out1) -> 0.04v2 +5v - u + j +140/1(In1)
  0.04v2 +5v - u + j +140/1(Out1) -> v + [0.04v2 +5v - u + j +140/1(In1)
  v + [0.04v2 +5v - u + j +140/1(Out1) -> u' switch/2(In2), v' switch/3(In3), v' switch/2(In2)
  a(bv-u)/1(Out1) -> u + a(bv-u)/2(In2)
  u + a(bv-u)/1(Out1) -> u' + d/2(In2), Delay8/1
  Delay8/1 -> u' switch/3(In3)
  Delay6/1 -> u' switch/1(In1)

== system ensembleSNN_simulink/izhiekvichNeuron7 ==
  J : Inport
  -65 : Constant  Value=-65
  0.04v2 +5v - u : Subsystem
  0.04v2 +5v - u + j +140 : Subsystem
  0.04v^2 : Subsystem
  0.04v^2 +5v : Subsystem
  140 : Constant  Value=140
  5v : Subsystem
  Constant1 : Constant  Value=5
  Constant2 : Constant  Value=0.04
  Delay1 : Delay  DelayLength=4
  Delay2 : Delay  DelayLength=1
  Delay3 : Delay  DelayLength=3
  Delay5 : Delay  DelayLength=1
  Delay6 : Delay
  Delay7 : Delay  DelayLength=7
  Delay8 : Delay  DelayLength=4
  a : Constant  Value=0.02
  a(bv-u) : Subsystem
  b : Constant  Value=0.2
  bv : Subsystem
  bv - u : Subsystem
  d : Constant  Value=8
  j + 140 : Subsystem
  u + a(bv-u) : Subsystem
  u' + d : Subsystem
  u' switch : Subsystem
  v + [0.04v2 +5v - u + j +140 : Subsystem
  v' switch : Subsystem
  v^2 : Subsystem
  voltage : Outport
  wires:
  d/1 -> u' + d/1(In1)
  Constant1/1 -> 5v/2(In2)
  Constant2/1 -> 0.04v^2/1(In1)
  140/1 -> j + 140/1(In1)
  -65/1 -> v' switch/1(In1)
  b/1 -> bv/1(In1)
  a/1 -> a(bv-u)/1(In1)
  5v/1(Out1) -> Delay5/1
  J/1 -> j + 140/2(J)
  j + 140/1(Out1) -> 0.04v2 +5v - u + j +140/2(J)
  u' + d/1(Out1) -> Delay6/1
  u' switch/1(Out1) -> Delay1/1, Delay3/1, Delay2/1
  Delay1/1 -> 0.04v2 +5v - u/2(In2)
  Delay2/1 -> bv - u/2(In2)
  Delay3/1 -> u + a(bv-u)/1(In1)
  v' switch/1(J) -> v^2/1(J), v^2/2(In2), 5v/1(J), bv/2(J), Delay7/1, voltage/1
  Delay7/1 -> v + [0.04v2 +5v - u + j +140/2(J)
  v^2/1(Out1) -> 0.04v^2/2(In2)
  Delay5/1 -> 0.04v^2 +5v/2(In2)
  bv/1(Out1) -> bv - u/1(In1)
  0.04v^2/1(Out1) -> 0.04v^2 +5v/1(In1)
  bv - u/1(Out1) -> a(bv-u)/2(In2)
  0.04v^2 +5v/1(Out1) -> 0.04v2 +5v - u/1(In1)
  0.04v2 +5v - u/1(Out1) -> 0.04v2 +5v - u + j +140/1(In1)
  0.04v2 +5v - u + j +140/1(Out1) -> v + [0.04v2 +5v - u + j +140/1(In1)
  v + [0.04v2 +5v - u + j +140/1(Out1) -> u' switch/2(In2), v' switch/3(In3), v' switch/2(In2)
  a(bv-u)/1(Out1) -> u + a(bv-u)/2(In2)
  u + a(bv-u)/1(Out1) -> u' + d/2(In2), Delay8/1
  Delay8/1 -> u' switch/3(In3)
  Delay6/1 -> u' switch/1(In1)

== system ensembleSNN_simulink/izhiekvichNeuron8 ==
  J : Inport
  -65 : Constant  Value=-65
  0.04v2 +5v - u : Subsystem
  0.04v2 +5v - u + j +140 : Subsystem
  0.04v^2 : Subsystem
  0.04v^2 +5v : Subsystem
  140 : Constant  Value=140
  5v : Subsystem
  Constant1 : Constant  Value=5
  Constant2 : Constant  Value=0.04
  Delay1 : Delay  DelayLength=4
  Delay2 : Delay  DelayLength=1
  Delay3 : Delay  DelayLength=3
  Delay5 : Delay  DelayLength=1
  Delay6 : Delay
  Delay7 : Delay  DelayLength=7
  Delay8 : Delay  DelayLength=4
  a : Constant  Value=0.02
  a(bv-u) : Subsystem
  b : Constant  Value=0.2
  bv : Subsystem
  bv - u : Subsystem
  d : Constant  Value=8
  j + 140 : Subsystem
  u + a(bv-u) : Subsystem
  u' + d : Subsystem
  u' switch : Subsystem
  v + [0.04v2 +5v - u + j +140 : Subsystem
  v' switch : Subsystem
  v^2 : Subsystem
  voltage : Outport
  wires:
  d/1 -> u' + d/1(In1)
  Constant1/1 -> 5v/2(In2)
  Constant2/1 -> 0.04v^2/1(In1)
  140/1 -> j + 140/1(In1)
  -65/1 -> v' switch/1(In1)
  b/1 -> bv/1(In1)
  a/1 -> a(bv-u)/1(In1)
  5v/1(Out1) -> Delay5/1
  J/1 -> j + 140/2(J)
  j + 140/1(Out1) -> 0.04v2 +5v - u + j +140/2(J)
  u' + d/1(Out1) -> Delay6/1
  u' switch/1(Out1) -> Delay1/1, Delay3/1, Delay2/1
  Delay1/1 -> 0.04v2 +5v - u/2(In2)
  Delay2/1 -> bv - u/2(In2)
  Delay3/1 -> u + a(bv-u)/1(In1)
  v' switch/1(J) -> v^2/1(J), v^2/2(In2), 5v/1(J), bv/2(J), Delay7/1, voltage/1
  Delay7/1 -> v + [0.04v2 +5v - u + j +140/2(J)
  v^2/1(Out1) -> 0.04v^2/2(In2)
  Delay5/1 -> 0.04v^2 +5v/2(In2)
  bv/1(Out1) -> bv - u/1(In1)
  0.04v^2/1(Out1) -> 0.04v^2 +5v/1(In1)
  bv - u/1(Out1) -> a(bv-u)/2(In2)
  0.04v^2 +5v/1(Out1) -> 0.04v2 +5v - u/1(In1)
  0.04v2 +5v - u/1(Out1) -> 0.04v2 +5v - u + j +140/1(In1)
  0.04v2 +5v - u + j +140/1(Out1) -> v + [0.04v2 +5v - u + j +140/1(In1)
  v + [0.04v2 +5v - u + j +140/1(Out1) -> u' switch/2(In2), v' switch/3(In3), v' switch/2(In2)
  a(bv-u)/1(Out1) -> u + a(bv-u)/2(In2)
  u + a(bv-u)/1(Out1) -> u' + d/2(In2), Delay8/1
  Delay8/1 -> u' switch/3(In3)
  Delay6/1 -> u' switch/1(In1)

== system ensembleSNN_simulink/izhiekvichNeuron9 ==
  J : Inport
  -65 : Constant  Value=-65
  0.04v2 +5v - u : Subsystem
  0.04v2 +5v - u + j +140 : Subsystem
  0.04v^2 : Subsystem
  0.04v^2 +5v : Subsystem
  140 : Constant  Value=140
  5v : Subsystem
  Constant1 : Constant  Value=5
  Constant2 : Constant  Value=0.04
  Delay1 : Delay  DelayLength=4
  Delay2 : Delay  DelayLength=1
  Delay3 : Delay  DelayLength=3
  Delay5 : Delay  DelayLength=1
  Delay6 : Delay
  Delay7 : Delay  DelayLength=7
  Delay8 : Delay  DelayLength=4
  a : Constant  Value=0.02
  a(bv-u) : Subsystem
  b : Constant  Value=0.2
  bv : Subsystem
  bv - u : Subsystem
  d : Constant  Value=8
  j + 140 : Subsystem
  u + a(bv-u) : Subsystem
  u' + d : Subsystem
  u' switch : Subsystem
  v + [0.04v2 +5v - u + j +140 : Subsystem
  v' switch : Subsystem
  v^2 : Subsystem
  voltage : Outport
  wires:
  d/1 -> u' + d/1(In1)
  Constant1/1 -> 5v/2(In2)
  Constant2/1 -> 0.04v^2/1(In1)
  140/1 -> j + 140/1(In1)
  -65/1 -> v' switch/1(In1)
  b/1 -> bv/1(In1)
  a/1 -> a(bv-u)/1(In1)
  5v/1(Out1) -> Delay5/1
  J/1 -> j + 140/2(J)
  j + 140/1(Out1) -> 0.04v2 +5v - u + j +140/2(J)
  u' + d/1(Out1) -> Delay6/1
  u' switch/1(Out1) -> Delay1/1, Delay3/1, Delay2/1
  Delay1/1 -> 0.04v2 +5v - u/2(In2)
  Delay2/1 -> bv - u/2(In2)
  Delay3/1 -> u + a(bv-u)/1(In1)
  v' switch/1(J) -> v^2/1(J), v^2/2(In2), 5v/1(J), bv/2(J), Delay7/1, voltage/1
  Delay7/1 -> v + [0.04v2 +5v - u + j +140/2(J)
  v^2/1(Out1) -> 0.04v^2/2(In2)
  Delay5/1 -> 0.04v^2 +5v/2(In2)
  bv/1(Out1) -> bv - u/1(In1)
  0.04v^2/1(Out1) -> 0.04v^2 +5v/1(In1)
  bv - u/1(Out1) -> a(bv-u)/2(In2)
  0.04v^2 +5v/1(Out1) -> 0.04v2 +5v - u/1(In1)
  0.04v2 +5v - u/1(Out1) -> 0.04v2 +5v - u + j +140/1(In1)
  0.04v2 +5v - u + j +140/1(Out1) -> v + [0.04v2 +5v - u + j +140/1(In1)
  v + [0.04v2 +5v - u + j +140/1(Out1) -> u' switch/2(In2), v' switch/3(In3), v' switch/2(In2)
  a(bv-u)/1(Out1) -> u + a(bv-u)/2(In2)
  u + a(bv-u)/1(Out1) -> u' + d/2(In2), Delay8/1
  Delay8/1 -> u' switch/3(In3)
  Delay6/1 -> u' switch/1(In1)

== system ensembleSNN_simulink/izhiekvichNeuron/0.04v2 +5v - u ==
  In1 : Inport
  In2 : Inport  Port=2
  Subtract : Sum  Inputs=+-
  Subtract Delay - 1 : Delay  DelayLength=1
  Out1 : Outport  VectorParamsAs1DForOutWhenUnconnected=on
  wires:
  In1/1 -> Subtract/1
  Subtract/1 -> Subtract Delay - 1/1
  Subtract Delay - 1/1 -> Out1/1
  In2/1 -> Subtract/2

== system ensembleSNN_simulink/izhiekvichNeuron/0.04v2 +5v - u + j +140 ==
  In1 : Inport
  J : Inport  Port=2
  Add : Sum
  Add Delay - 2 : Delay
  Out1 : Outport  VectorParamsAs1DForOutWhenUnconnected=on
  wires:
  Add Delay - 2/1 -> Out1/1
  Add/1 -> Add Delay - 2/1
  In1/1 -> Add/1
  J/1 -> Add/2

== system ensembleSNN_simulink/izhiekvichNeuron/0.04v^2 ==
  In1 : Inport
  In2 : Inport  Port=2
  Mult Delay - 1 : Delay  DelayLength=1
  Product1 : Product
  Out1 : Outport  VectorParamsAs1DForOutWhenUnconnected=on
  wires:
  Product1/1 -> Mult Delay - 1/1
  Mult Delay - 1/1 -> Out1/1
  In2/1 -> Product1/2
  In1/1 -> Product1/1

== system ensembleSNN_simulink/izhiekvichNeuron/0.04v^2 +5v ==
  In1 : Inport
  In2 : Inport  Port=2
  Add : Sum
  Add Delay - 2 : Delay
  Out1 : Outport  VectorParamsAs1DForOutWhenUnconnected=on
  wires:
  Add Delay - 2/1 -> Out1/1
  Add/1 -> Add Delay - 2/1
  In1/1 -> Add/1
  In2/1 -> Add/2

== system ensembleSNN_simulink/izhiekvichNeuron/5v ==
  J : Inport
  In2 : Inport  Port=2
  Mult Delay - 1 : Delay  DelayLength=1
  Product1 : Product
  Out1 : Outport  VectorParamsAs1DForOutWhenUnconnected=on
  wires:
  Product1/1 -> Mult Delay - 1/1
  Mult Delay - 1/1 -> Out1/1
  In2/1 -> Product1/2
  J/1 -> Product1/1

== system ensembleSNN_simulink/izhiekvichNeuron/a(bv-u) ==
  In1 : Inport
  In2 : Inport  Port=2
  Mult Delay - 1 : Delay  DelayLength=1
  Product1 : Product
  Out1 : Outport  VectorParamsAs1DForOutWhenUnconnected=on
  wires:
  Product1/1 -> Mult Delay - 1/1
  Mult Delay - 1/1 -> Out1/1
  In2/1 -> Product1/2
  In1/1 -> Product1/1

== system ensembleSNN_simulink/izhiekvichNeuron/bv ==
  In1 : Inport
  J : Inport  Port=2
  Mult Delay - 1 : Delay  DelayLength=1
  Product1 : Product
  Out1 : Outport  VectorParamsAs1DForOutWhenUnconnected=on
  wires:
  Product1/1 -> Mult Delay - 1/1
  Mult Delay - 1/1 -> Out1/1
  J/1 -> Product1/2
  In1/1 -> Product1/1

== system ensembleSNN_simulink/izhiekvichNeuron/bv - u ==
  In1 : Inport
  In2 : Inport  Port=2
  Subtract : Sum  Inputs=+-
  Subtract Delay - 1 : Delay  DelayLength=1
  Out1 : Outport  VectorParamsAs1DForOutWhenUnconnected=on
  wires:
  In1/1 -> Subtract/1
  Subtract/1 -> Subtract Delay - 1/1
  Subtract Delay - 1/1 -> Out1/1
  In2/1 -> Subtract/2

== system ensembleSNN_simulink/izhiekvichNeuron/j + 140 ==
  In1 : Inport
  J : Inport  Port=2
  Add : Sum
  Add Delay - 2 : Delay
  Out1 : Outport  VectorParamsAs1DForOutWhenUnconnected=on
  wires:
  Add Delay - 2/1 -> Out1/1
  Add/1 -> Add Delay - 2/1
  In1/1 -> Add/1
  J/1 -> Add/2

== system ensembleSNN_simulink/izhiekvichNeuron/u + a(bv-u) ==
  In1 : Inport
  In2 : Inport  Port=2
  Add : Sum
  Add Delay - 2 : Delay
  Out1 : Outport  VectorParamsAs1DForOutWhenUnconnected=on
  wires:
  Add Delay - 2/1 -> Out1/1
  Add/1 -> Add Delay - 2/1
  In1/1 -> Add/1
  In2/1 -> Add/2

== system ensembleSNN_simulink/izhiekvichNeuron/u' + d ==
  In1 : Inport
  In2 : Inport  Port=2
  Add : Sum
  Add Delay - 2 : Delay
  Out1 : Outport  VectorParamsAs1DForOutWhenUnconnected=on
  wires:
  Add Delay - 2/1 -> Out1/1
  Add/1 -> Add Delay - 2/1
  In1/1 -> Add/1
  In2/1 -> Add/2

== system ensembleSNN_simulink/izhiekvichNeuron/u' switch ==
  In1 : Inport
  In2 : Inport  Port=2
  In3 : Inport  Port=3
  Switch Delay - 3 : Delay  DelayLength=3
  Switch4 : Switch  Criteria=u2 > Threshold  Threshold=30
  Out1 : Outport  VectorParamsAs1DForOutWhenUnconnected=on
  wires:
  In2/1 -> Switch4/2
  Switch4/1 -> Switch Delay - 3/1
  In1/1 -> Switch4/1
  Switch Delay - 3/1 -> Out1/1
  In3/1 -> Switch4/3

== system ensembleSNN_simulink/izhiekvichNeuron/v + [0.04v2 +5v - u + j +140 ==
  In1 : Inport
  J : Inport  Port=2
  Add : Sum
  Add Delay - 2 : Delay
  Out1 : Outport  VectorParamsAs1DForOutWhenUnconnected=on
  wires:
  Add Delay - 2/1 -> Out1/1
  Add/1 -> Add Delay - 2/1
  In1/1 -> Add/1
  J/1 -> Add/2

== system ensembleSNN_simulink/izhiekvichNeuron/v' switch ==
  In1 : Inport
  In2 : Inport  Port=2
  In3 : Inport  Port=3
  Switch Delay - 3 : Delay  DelayLength=3
  Switch4 : Switch  Criteria=u2 > Threshold  Threshold=30
  J : Outport  VectorParamsAs1DForOutWhenUnconnected=on
  wires:
  In2/1 -> Switch4/2
  Switch4/1 -> Switch Delay - 3/1
  In1/1 -> Switch4/1
  Switch Delay - 3/1 -> J/1
  In3/1 -> Switch4/3

== system ensembleSNN_simulink/izhiekvichNeuron/v^2 ==
  J : Inport
  In2 : Inport  Port=2
  Mult Delay - 2 : Delay  DelayLength=1
  Product1 : Product
  Out1 : Outport  VectorParamsAs1DForOutWhenUnconnected=on
  wires:
  Product1/1 -> Mult Delay - 2/1
  In2/1 -> Product1/2
  J/1 -> Product1/1
  Mult Delay - 2/1 -> Out1/1

== system ensembleSNN_simulink/izhiekvichNeuron1/0.04v2 +5v - u ==
  In1 : Inport
  In2 : Inport  Port=2
  Subtract : Sum  Inputs=+-
  Subtract Delay - 1 : Delay  DelayLength=1
  Out1 : Outport  VectorParamsAs1DForOutWhenUnconnected=on
  wires:
  In1/1 -> Subtract/1
  Subtract/1 -> Subtract Delay - 1/1
  Subtract Delay - 1/1 -> Out1/1
  In2/1 -> Subtract/2

== system ensembleSNN_simulink/izhiekvichNeuron1/0.04v2 +5v - u + j +140 ==
  In1 : Inport
  J : Inport  Port=2
  Add : Sum
  Add Delay - 2 : Delay
  Out1 : Outport  VectorParamsAs1DForOutWhenUnconnected=on
  wires:
  Add Delay - 2/1 -> Out1/1
  Add/1 -> Add Delay - 2/1
  In1/1 -> Add/1
  J/1 -> Add/2

== system ensembleSNN_simulink/izhiekvichNeuron1/0.04v^2 ==
  In1 : Inport
  In2 : Inport  Port=2
  Mult Delay - 1 : Delay  DelayLength=1
  Product1 : Product
  Out1 : Outport  VectorParamsAs1DForOutWhenUnconnected=on
  wires:
  Product1/1 -> Mult Delay - 1/1
  Mult Delay - 1/1 -> Out1/1
  In2/1 -> Product1/2
  In1/1 -> Product1/1

== system ensembleSNN_simulink/izhiekvichNeuron1/0.04v^2 +5v ==
  In1 : Inport
  In2 : Inport  Port=2
  Add : Sum
  Add Delay - 2 : Delay
  Out1 : Outport  VectorParamsAs1DForOutWhenUnconnected=on
  wires:
  Add Delay - 2/1 -> Out1/1
  Add/1 -> Add Delay - 2/1
  In1/1 -> Add/1
  In2/1 -> Add/2

== system ensembleSNN_simulink/izhiekvichNeuron1/5v ==
  J : Inport
  In2 : Inport  Port=2
  Mult Delay - 1 : Delay  DelayLength=1
  Product1 : Product
  Out1 : Outport  VectorParamsAs1DForOutWhenUnconnected=on
  wires:
  Product1/1 -> Mult Delay - 1/1
  Mult Delay - 1/1 -> Out1/1
  In2/1 -> Product1/2
  J/1 -> Product1/1

== system ensembleSNN_simulink/izhiekvichNeuron1/a(bv-u) ==
  In1 : Inport
  In2 : Inport  Port=2
  Mult Delay - 1 : Delay  DelayLength=1
  Product1 : Product
  Out1 : Outport  VectorParamsAs1DForOutWhenUnconnected=on
  wires:
  Product1/1 -> Mult Delay - 1/1
  Mult Delay - 1/1 -> Out1/1
  In2/1 -> Product1/2
  In1/1 -> Product1/1

== system ensembleSNN_simulink/izhiekvichNeuron1/bv ==
  In1 : Inport
  J : Inport  Port=2
  Mult Delay - 1 : Delay  DelayLength=1
  Product1 : Product
  Out1 : Outport  VectorParamsAs1DForOutWhenUnconnected=on
  wires:
  Product1/1 -> Mult Delay - 1/1
  Mult Delay - 1/1 -> Out1/1
  J/1 -> Product1/2
  In1/1 -> Product1/1

== system ensembleSNN_simulink/izhiekvichNeuron1/bv - u ==
  In1 : Inport
  In2 : Inport  Port=2
  Subtract : Sum  Inputs=+-
  Subtract Delay - 1 : Delay  DelayLength=1
  Out1 : Outport  VectorParamsAs1DForOutWhenUnconnected=on
  wires:
  In1/1 -> Subtract/1
  Subtract/1 -> Subtract Delay - 1/1
  Subtract Delay - 1/1 -> Out1/1
  In2/1 -> Subtract/2

== system ensembleSNN_simulink/izhiekvichNeuron1/j + 140 ==
  In1 : Inport
  J : Inport  Port=2
  Add : Sum
  Add Delay - 2 : Delay
  Out1 : Outport  VectorParamsAs1DForOutWhenUnconnected=on
  wires:
  Add Delay - 2/1 -> Out1/1
  Add/1 -> Add Delay - 2/1
  In1/1 -> Add/1
  J/1 -> Add/2

== system ensembleSNN_simulink/izhiekvichNeuron1/u + a(bv-u) ==
  In1 : Inport
  In2 : Inport  Port=2
  Add : Sum
  Add Delay - 2 : Delay
  Out1 : Outport  VectorParamsAs1DForOutWhenUnconnected=on
  wires:
  Add Delay - 2/1 -> Out1/1
  Add/1 -> Add Delay - 2/1
  In1/1 -> Add/1
  In2/1 -> Add/2

== system ensembleSNN_simulink/izhiekvichNeuron1/u' + d ==
  In1 : Inport
  In2 : Inport  Port=2
  Add : Sum
  Add Delay - 2 : Delay
  Out1 : Outport  VectorParamsAs1DForOutWhenUnconnected=on
  wires:
  Add Delay - 2/1 -> Out1/1
  Add/1 -> Add Delay - 2/1
  In1/1 -> Add/1
  In2/1 -> Add/2

== system ensembleSNN_simulink/izhiekvichNeuron1/u' switch ==
  In1 : Inport
  In2 : Inport  Port=2
  In3 : Inport  Port=3
  Switch Delay - 3 : Delay  DelayLength=3
  Switch4 : Switch  Criteria=u2 > Threshold  Threshold=30
  Out1 : Outport  VectorParamsAs1DForOutWhenUnconnected=on
  wires:
  In2/1 -> Switch4/2
  Switch4/1 -> Switch Delay - 3/1
  In1/1 -> Switch4/1
  Switch Delay - 3/1 -> Out1/1
  In3/1 -> Switch4/3

== system ensembleSNN_simulink/izhiekvichNeuron1/v + [0.04v2 +5v - u + j +140 ==
  In1 : Inport
  J : Inport  Port=2
  Add : Sum
  Add Delay - 2 : Delay
  Out1 : Outport  VectorParamsAs1DForOutWhenUnconnected=on
  wires:
  Add Delay - 2/1 -> Out1/1
  Add/1 -> Add Delay - 2/1
  In1/1 -> Add/1
  J/1 -> Add/2

== system ensembleSNN_simulink/izhiekvichNeuron1/v' switch ==
  In1 : Inport
  In2 : Inport  Port=2
  In3 : Inport  Port=3
  Switch Delay - 3 : Delay  DelayLength=3
  Switch4 : Switch  Criteria=u2 > Threshold  Threshold=30
  J : Outport  VectorParamsAs1DForOutWhenUnconnected=on
  wires:
  In2/1 -> Switch4/2
  Switch4/1 -> Switch Delay - 3/1
  In1/1 -> Switch4/1
  Switch Delay - 3/1 -> J/1
  In3/1 -> Switch4/3

== system ensembleSNN_simulink/izhiekvichNeuron1/v^2 ==
  J : Inport
  In2 : Inport  Port=2
  Mult Delay - 2 : Delay  DelayLength=1
  Product1 : Product
  Out1 : Outport  VectorParamsAs1DForOutWhenUnconnected=on
  wires:
  Product1/1 -> Mult Delay - 2/1
  In2/1 -> Product1/2
  J/1 -> Product1/1
  Mult Delay - 2/1 -> Out1/1

== system ensembleSNN_simulink/izhiekvichNeuron10/0.04v2 +5v - u ==
  In1 : Inport
  In2 : Inport  Port=2
  Subtract : Sum  Inputs=+-
  Subtract Delay - 1 : Delay  DelayLength=1
  Out1 : Outport  VectorParamsAs1DForOutWhenUnconnected=on
  wires:
  In1/1 -> Subtract/1
  Subtract/1 -> Subtract Delay - 1/1
  Subtract Delay - 1/1 -> Out1/1
  In2/1 -> Subtract/2

== system ensembleSNN_simulink/izhiekvichNeuron10/0.04v2 +5v - u + j +140 ==
  In1 : Inport
  J : Inport  Port=2
  Add : Sum
  Add Delay - 2 : Delay
  Out1 : Outport  VectorParamsAs1DForOutWhenUnconnected=on
  wires:
  Add Delay - 2/1 -> Out1/1
  Add/1 -> Add Delay - 2/1
  In1/1 -> Add/1
  J/1 -> Add/2

== system ensembleSNN_simulink/izhiekvichNeuron10/0.04v^2 ==
  In1 : Inport
  In2 : Inport  Port=2
  Mult Delay - 1 : Delay  DelayLength=1
  Product1 : Product
  Out1 : Outport  VectorParamsAs1DForOutWhenUnconnected=on
  wires:
  Product1/1 -> Mult Delay - 1/1
  Mult Delay - 1/1 -> Out1/1
  In2/1 -> Product1/2
  In1/1 -> Product1/1

== system ensembleSNN_simulink/izhiekvichNeuron10/0.04v^2 +5v ==
  In1 : Inport
  In2 : Inport  Port=2
  Add : Sum
  Add Delay - 2 : Delay
  Out1 : Outport  VectorParamsAs1DForOutWhenUnconnected=on
  wires:
  Add Delay - 2/1 -> Out1/1
  Add/1 -> Add Delay - 2/1
  In1/1 -> Add/1
  In2/1 -> Add/2

== system ensembleSNN_simulink/izhiekvichNeuron10/5v ==
  J : Inport
  In2 : Inport  Port=2
  Mult Delay - 1 : Delay  DelayLength=1
  Product1 : Product
  Out1 : Outport  VectorParamsAs1DForOutWhenUnconnected=on
  wires:
  Product1/1 -> Mult Delay - 1/1
  Mult Delay - 1/1 -> Out1/1
  In2/1 -> Product1/2
  J/1 -> Product1/1

== system ensembleSNN_simulink/izhiekvichNeuron10/a(bv-u) ==
  In1 : Inport
  In2 : Inport  Port=2
  Mult Delay - 1 : Delay  DelayLength=1
  Product1 : Product
  Out1 : Outport  VectorParamsAs1DForOutWhenUnconnected=on
  wires:
  Product1/1 -> Mult Delay - 1/1
  Mult Delay - 1/1 -> Out1/1
  In2/1 -> Product1/2
  In1/1 -> Product1/1

== system ensembleSNN_simulink/izhiekvichNeuron10/bv ==
  In1 : Inport
  J : Inport  Port=2
  Mult Delay - 1 : Delay  DelayLength=1
  Product1 : Product
  Out1 : Outport  VectorParamsAs1DForOutWhenUnconnected=on
  wires:
  Product1/1 -> Mult Delay - 1/1
  Mult Delay - 1/1 -> Out1/1
  J/1 -> Product1/2
  In1/1 -> Product1/1

== system ensembleSNN_simulink/izhiekvichNeuron10/bv - u ==
  In1 : Inport
  In2 : Inport  Port=2
  Subtract : Sum  Inputs=+-
  Subtract Delay - 1 : Delay  DelayLength=1
  Out1 : Outport  VectorParamsAs1DForOutWhenUnconnected=on
  wires:
  In1/1 -> Subtract/1
  Subtract/1 -> Subtract Delay - 1/1
  Subtract Delay - 1/1 -> Out1/1
  In2/1 -> Subtract/2

== system ensembleSNN_simulink/izhiekvichNeuron10/j + 140 ==
  In1 : Inport
  J : Inport  Port=2
  Add : Sum
  Add Delay - 2 : Delay
  Out1 : Outport  VectorParamsAs1DForOutWhenUnconnected=on
  wires:
  Add Delay - 2/1 -> Out1/1
  Add/1 -> Add Delay - 2/1
  In1/1 -> Add/1
  J/1 -> Add/2

== system ensembleSNN_simulink/izhiekvichNeuron10/u + a(bv-u) ==
  In1 : Inport
  In2 : Inport  Port=2
  Add : Sum
  Add Delay - 2 : Delay
  Out1 : Outport  VectorParamsAs1DForOutWhenUnconnected=on
  wires:
  Add Delay - 2/1 -> Out1/1
  Add/1 -> Add Delay - 2/1
  In1/1 -> Add/1
  In2/1 -> Add/2

== system ensembleSNN_simulink/izhiekvichNeuron10/u' + d ==
  In1 : Inport
  In2 : Inport  Port=2
  Add : Sum
  Add Delay - 2 : Delay
  Out1 : Outport  VectorParamsAs1DForOutWhenUnconnected=on
  wires:
  Add Delay - 2/1 -> Out1/1
  Add/1 -> Add Delay - 2/1
  In1/1 -> Add/1
  In2/1 -> Add/2
